simulink model "landing_model4"  (R2020a)
settings: Solver=ode3  StartTime=0.0  StopTime=Inf  RelTol=1e-3  EnableMultiTasking=on
libraries: dspsigops x3, visionstatistics x1, visionanalysis x1, simulink x1, embdlinuxlib x1
settings Model: FPTRunName=Active  ExtModeTrigDuration=2  Creator=ianli  LastModifiedBy=taniafolabi
settings SolverCC: PositivePriorityOrder=on
settings DataIOCC: LimitDataPoints=on  SaveFormat=Array
settings OptimizationCC: ExpressionDepthLimit=2147483647  LifeSpan=Inf  MaxStackSize=64
settings DebuggingCC: UnderspecifiedInitializationDetection=Classic  MergeDetectMultiDrivingBlocksExec=none  FcnCallInpInsideContextMsg=warning  AllowSymbolicDim=off  StateNameClashWarn=warning  SFUnexpectedBacktrackingDiag=warning  SFNoUnconditionalDefaultTransitionDiag=warning  SFExecutionAtInitializationDiag=none  ArithmeticOperatorsInVariantConditions=warning
settings HardwareCC: ProdBitPerPointer=32  ProdBitPerSizeT=32  ProdBitPerPtrDiffT=32  ProdLargestAtomicInteger=Long  ProdLargestAtomicFloat=Double  ProdWordSize=32  ProdHWDeviceType=ARM Compatible->ARM Cortex  UseEmbeddedCoderFeatures=off
settings ModelReferenceCC: PropagateSignalLabelsOutOfModel=off
settings SFSimCC: SimUseLocalCustomCode=off  CustomCodeUndefinedFunction=UseInterfaceOnly
settings RTWCC: SystemTargetFile=ert.tlc  HardwareBoard=Raspberry Pi  TemplateMakefile=ert_default_tmf  GenerateReport=on  RTWVerbose=off  RTWUseLocalCustomCode=off  Toolchain=GNU GCC Raspberry Pi  BuildConfiguration=Faster Runs  LaunchReport=on
settings CodeAppCC: ForceParamTrailComments=on  OperatorAnnotations=on  StateflowObjectComments=on  MATLABSourceComments=on
settings ERTTargetCC: MultiwordLength=2048  ERTCustomFileBanners=off  SupportContinuousTime=on  SupportNonInlinedSFcns=on  RemoveResetFunc=off  SupportVariableSizeSignals=on  ModelStepFunctionPrototypeControlCompliant=off
settings ConfigComp: CovMetricSettings=dw  CovHtmlReporting=on  CovSaveCumulativeToWorkspaceVar=on  CovSaveSingleToWorkspaceVar=on  CovExternalEMLEnable=off  CovSFcnEnable=off

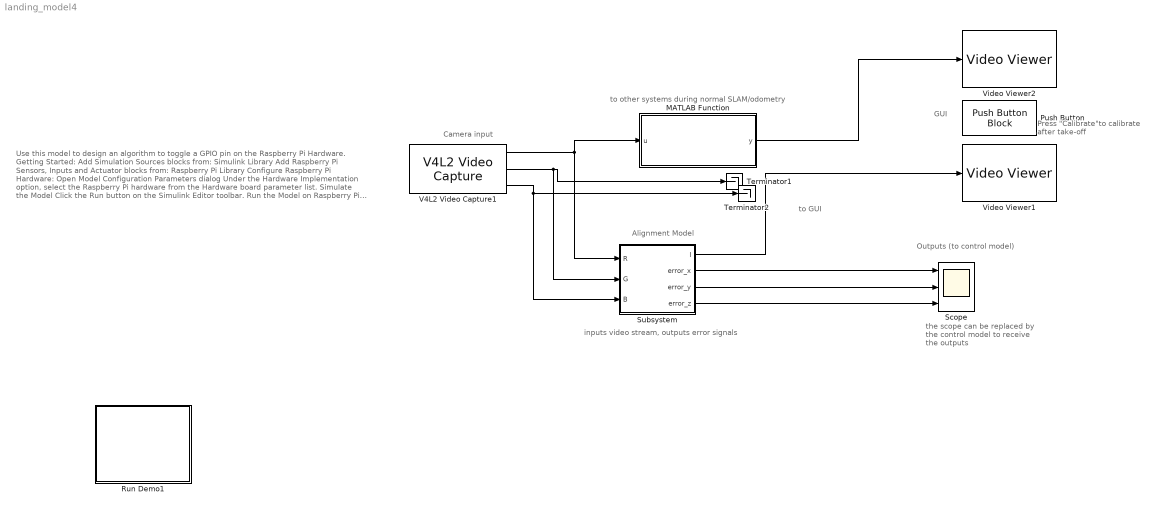
== system landing_model4 ==
  note: Outputs (to control model)
  note: inputs video stream, outputs error signals
  note: Camera input
  note: Alignment Model
  note: Press "Calibrate"to calibrate after take-off
  note: to GUI
  note: the scope can be replaced by the control model to receive the outputs
  note: GUI
  note: to other systems during normal SLAM/odometry
  note: Use this model to design an algorithm to toggle a GPIO pin on the Raspberry Pi Hardware.
      |
      | Getting Started:
      |
      | Add Simulation Sources blocks from:
      | Simulink Library
      | Add Raspberry Pi Sensors, Inputs and Actuator blocks from:
      | Raspberry Pi Library
      |
      | Configure Raspberry Pi Hardware:
      |
      | Open Model Configuration Parameters dialog
      | Under the Hardware Implementation option, select the Raspberry Pi hardware from the Hardware board parameter list.
      |
      | Simulate the Model
      |
      | Click the Run button on the Simulink Editor toolbar.
      |
      | Run the Model on Raspberry Pi Hardware
      |
      | In the Hardware tab, click Build, Deploy & Start
      |
      | Other Things to Try:
      |
      | Create and run a model that repeatedly brightens and dims an LED. Hint: Use PWM block as an Raspberry Pi actuator.
  MATLAB Function : MATLAB Function  TreatAsAtomicUnit=on
  Push Button : PushButtonBlock  ButtonText=Callibrate
  Run Demo1 : Subsystem  Description=Controls host-side RTDX processing.
      mask Display: pic=imread('raspberrypiBuildDeployAndStart.png');image(pic);
  Scope : Scope  NumInputPorts=3
  Subsystem : Subsystem
  Terminator1 : Terminator
  Terminator2 : Terminator
  V4L2 Video Capture1 : embdlinuxlib/V4L2 Video Capture  m_devName='/dev/video0'  roi=[0, 0, 640, 480]  imSizeSelection=640x480  imSize=[640, 480]  pixelFormat=RGB  pixelOrder=Planar  sampleTime=1/10  simOutput=Colorbars  blockPlatform=Raspberry Pi
      settings: SourceProductBaseCode=SC_BEAGLEBONE_BLUE,RASPPI
  Video Viewer1 : VideoViewer  FigPos=[375 586 530.4 373.6]
  Video Viewer2 : VideoViewer  FigPos=[375 586 530.4 373.6]
  wires:
  Subsystem/1(I) -> Video Viewer1/1
  Subsystem/2(error_x) -> Scope/1
  Subsystem/3(error_y) -> Scope/2
  Subsystem/4(error_z) -> Scope/3
  V4L2 Video Capture1/2 -> Subsystem/2(G), Terminator1/1
  V4L2 Video Capture1/3 -> Subsystem/3(B), Terminator2/1
  V4L2 Video Capture1/1 -> MATLAB Function/1(u), Subsystem/1(R)
  MATLAB Function/1(y) -> Video Viewer2/1
  ? -> ?

== system landing_model4/Run Demo1 ==

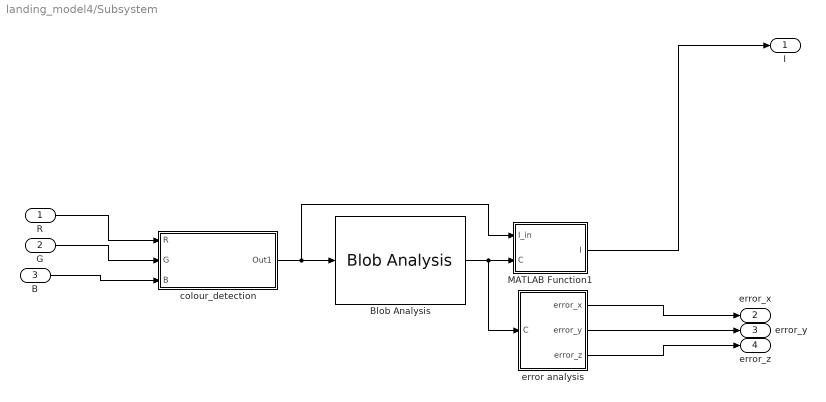
== system landing_model4/Subsystem ==
  R : Inport
  G : Inport  Port=2
  B : Inport  Port=3
  Blob Analysis : visionstatistics/Blob Analysis  Tag=vipblks_row_conv  area=off  centroid=on  bBox=off  majorAxis=off  minorAxis=off  angle=off  eccentricity=off  equivDiameterSq=off  extent=off  perimeter=off  outDT=double  conn=8  isLabel=off  maxBlobs=3  warnIfNumBlobsExceeded=on  isCount=off  useMinArea=off  minArea=0  useMaxArea=off  maxArea=intmax('uint32')  excludeBorderBlob=off  isOutVarDim=off  isFill=on  fillValues=-1  roundingMode=Floor  overflowMode=off  prodOutputMode=Binary point scaling  prodOutputWordLength=32  prodOutputFracLength=16  accumMode=Binary point scaling  accumWordLength=32  accumFracLength=0  outputMode=Binary point scaling  outputWordLength=32  outputFracLength=16  firstCoeffMode=Binary point scaling  firstCoeffWordLength=16  firstCoeffFracLength=14  secondCoeffMode=Binary point scaling  secondCoeffWordLength=32  secondCoeffFracLength=16
  MATLAB Function1 : MATLAB Function  TreatAsAtomicUnit=on
  colour_detection : Subsystem
  error analysis : Subsystem
  I : Outport
  error_x : Outport  Port=2
  error_y : Outport  Port=3
  error_z : Outport  Port=4
  wires:
  Blob Analysis/1 -> error analysis/1(C), MATLAB Function1/2(C)
  colour_detection/1(Out1) -> Blob Analysis/1, MATLAB Function1/1(I_in)
  error analysis/1(error_x) -> error_x/1
  MATLAB Function1/1(I) -> I/1
  error analysis/2(error_y) -> error_y/1
  error analysis/3(error_z) -> error_z/1
  R/1 -> colour_detection/1(R)
  G/1 -> colour_detection/2(G)
  B/1 -> colour_detection/3(B)

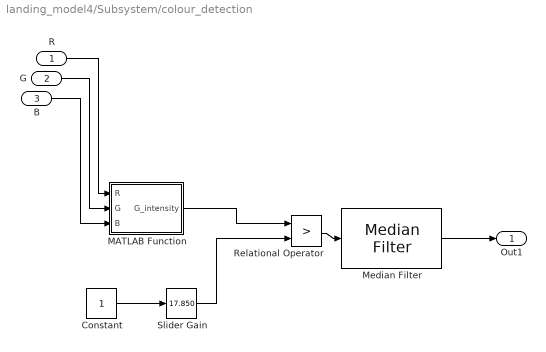
== system landing_model4/Subsystem/colour_detection ==
  R : Inport
  G : Inport  Port=2
  B : Inport  Port=3
  Constant : Constant
  MATLAB Function : MATLAB Function  TreatAsAtomicUnit=on
  Median Filter : visionanalysis/Median Filter  nghbood=[3 3]  outSize=Same as input port I  padType=Constant  padSrc=Specify via dialog  padVal=0  roundingMode=Floor  overflowMode=off
      settings: SourceProductBaseCode=VP
  Relational Operator : RelationalOperator  Operator=>  OutDataTypeStr=boolean  RndMeth=Simplest
  Slider Gain : simulink/Math Operations/Slider Gain  gain=17.850  low=0  high=255
  Out1 : Outport
  wires:
  Slider Gain/1 -> Relational Operator/2
  Constant/1 -> Slider Gain/1
  MATLAB Function/1(G_intensity) -> Relational Operator/1
  G/1 -> MATLAB Function/2(G)
  B/1 -> MATLAB Function/3(B)
  Median Filter/1 -> Out1/1
  R/1 -> MATLAB Function/1(R)
  Relational Operator/1 -> Median Filter/1

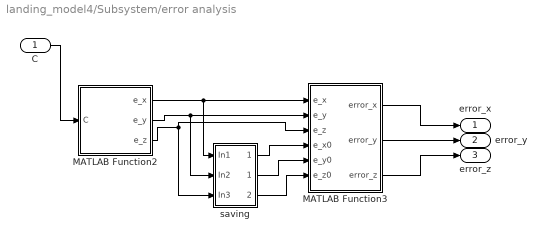
== system landing_model4/Subsystem/error analysis ==
  C : Inport
  MATLAB Function2 : MATLAB Function  TreatAsAtomicUnit=on
  MATLAB Function3 : MATLAB Function  TreatAsAtomicUnit=on
  saving : Subsystem
  error_x : Outport
  error_y : Outport  Port=2
  error_z : Outport  Port=3
  wires:
  MATLAB Function2/2(e_y) -> MATLAB Function3/2(e_y), saving/2(In2)
  MATLAB Function2/1(e_x) -> saving/1(In1), MATLAB Function3/1(e_x)
  saving/3(" 2") -> MATLAB Function3/6(e_z0)
  saving/2(" 1") -> MATLAB Function3/5(e_y0)
  MATLAB Function2/3(e_z) -> MATLAB Function3/3(e_z), saving/3(In3)
  saving/1(" ") -> MATLAB Function3/4(e_x0)
  MATLAB Function3/1(error_x) -> error_x/1
  MATLAB Function3/3(error_z) -> error_z/1
  MATLAB Function3/2(error_y) -> error_y/1
  C/1 -> MATLAB Function2/1(C)

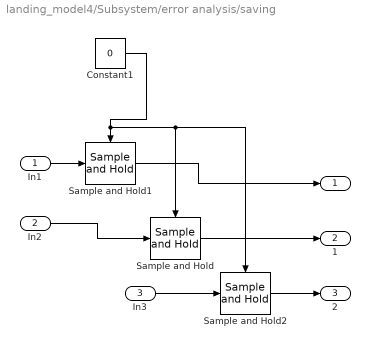
== system landing_model4/Subsystem/error analysis/saving ==
  In1 : Inport
  In2 : Inport  Port=2
  In3 : Inport  Port=3
  Constant1 : Constant  Value=0
  Sample and Hold : dspsigops/Sample and Hold  trig=Rising edge  initCond=0  latchinput=off
  Sample and Hold1 : dspsigops/Sample and Hold  trig=Rising edge  initCond=0  latchinput=off
  Sample and Hold2 : dspsigops/Sample and Hold  trig=Rising edge  initCond=0  latchinput=off
  " " : Outport
  " 1" : Outport  Port=2
  " 2" : Outport  Port=3
  wires:
  Sample and Hold1/1 -> " "/1
  In1/1 -> Sample and Hold1/1
  In2/1 -> Sample and Hold/1
  Sample and Hold/1 -> " 1"/1
  Sample and Hold2/1 -> " 2"/1
  In3/1 -> Sample and Hold2/1
  Constant1/1 -> Sample and Hold2/Trigger, Sample and Hold/Trigger, Sample and Hold1/Trigger

== matlab function landing_model4/Subsystem/MATLAB Function1 ==
  data: I_in input; I output; C input
function I = fcn(I_in,C)
w = length(I_in(1,:));
h = length(I_in(:,1));
I = I_in;
for i = 1:length(C)
I(:,C(i,1)) = ones(h,1); % vertical bars
I(C(i,2),:) = ones(1,w); % horizontal bars
end

== matlab function landing_model4/Subsystem/colour_detection/MATLAB Function ==
  data: R input; G_intensity output; G input; B input
function G_intensity  = fcn(R,G,B)

G_intensity = G - R./2 - B./2;

== matlab function landing_model4/Subsystem/error analysis/MATLAB Function2 ==
  data: C input; e_x output; e_y output; e_z output
function [e_x, e_y, e_z] = distances(C) % note everything is in pixels

% input C gives a 3-by-2 matrix in in the form [x1 y1 ; x2 y2 ; x3 y3] of
% the coordinates of the centroids
% (possible input that can be obtained from blob analysis is also blob area
% which can be used to identify the different blobs)
if length(C)==3
    C_sorted = sortrows(C); % sort so rows 1-3 correspond to blobs from L-R
    % NB blob 1,3 are the back markers, blob 3 is the front marker
    e_x = (C_sorted(3,1)+C_sorted(2,1))/2-C_sorted(2,1); %+ve error - too far right
    e_z = (C_sorted(3,2)+C_sorted(2,2))/2-C_sorted(2,2); %+ve error - too high
    e_y = (C_sorted(3,1)-C_sorted(1,1)); % relative distance between poles in pixels
end

== matlab function landing_model4/Subsystem/error analysis/MATLAB Function3 ==
  data: e_x input; e_y input; error_x output; error_y output; e_z input; e_x0 input; e_y0 input; e_z0 input; error_z output
function [error_x,error_y,error_z] = fcn(e_x,e_y,e_z,e_x0,e_y0,e_z0)

error_x = e_x-e_x0;
error_z = e_z-e_z0;
error_y = e_y-e_y0;

== matlab function landing_model4/MATLAB Function ==
  data: u input; y output
function y = PedestrianTracking(u)
[obj, tracks, full, FrameWithTracker] = PedestrianTracker();
objs = obj;
trackss = tracks;
y = [full, FrameWithTracker];
